simulink model "SchmittTriggers_mod"  (R2018b)
settings: Solver=FixedStepAuto  StartTime=0.0  StopTime=tstop  FixedStep=dt  RelTol=1e-3
values from neighbouring files (symbols this model uses):
  A = 5    [SchmittTriggers_data.m]
  f = 20    [SchmittTriggers_data.m]
  Us1 = 1    [SchmittTriggers_data.m]
  Usoff = -1    [SchmittTriggers_data.m]
  Uson = 1    [SchmittTriggers_data.m]
  Ustor = 3    [SchmittTriggers_data.m]
settings Model: Creator=Peter  LastModifiedBy=Peter

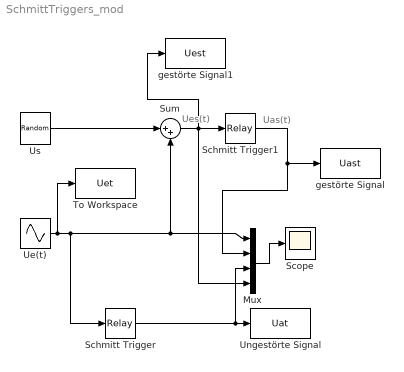
== system SchmittTriggers_mod ==
  note: Uas(t)
  note: Ues(t)
  Mux : Mux
  Schmitt Trigger : Relay  OnSwitchValue=Uson  OffSwitchValue=Usoff  OnOutputValue=Uamax  OffOutputValue=Uamin
  Schmitt Trigger1 : Relay  OnSwitchValue=Us1  OffSwitchValue=-Us1  OnOutputValue=Uamax  OffOutputValue=Uamin
  Scope : Scope
  Sum : Sum  Inputs=|++
  To Workspace : ToWorkspace  VariableName=Uet  SampleTime=-1
  "Ue(t) " : Sin  Amplitude=A  Frequency=2*pi*f  SampleTime=0
  Ungestörte Signal : ToWorkspace  VariableName=Uat  SampleTime=-1
  "Us " : UniformRandomNumber  Minimum=-Ustor  Maximum=Ustor  SampleTime=0
  gestörte Signal : ToWorkspace  VariableName=Uast  SampleTime=-1
  gestörte Signal1 : ToWorkspace  VariableName=Uest  SampleTime=-1
  wires:
  "Ue(t) "/1 -> To Workspace/1, Schmitt Trigger/1, Sum/2, Mux/1
  Schmitt Trigger/1 -> Mux/3, Ungestörte Signal/1
  Mux/1 -> Scope/1
  "Us "/1 -> Sum/1
  Sum/1 -> gestörte Signal1/1, Mux/4, Schmitt Trigger1/1
  Schmitt Trigger1/1 -> gestörte Signal/1, Mux/2
